simulink model "RTOS_Mail_blocking_Blinky"  (R2016b)
settings: Solver=FixedStepDiscrete  StartTime=0.0  StopTime=10.0  FixedStep=1e-3  RelTol=1e-3
libraries: mbed_lib x6
settings Model: MbedPath=E:\GitSynology\mbed_target\targets\NUCLEO_F303RE  Creator=oh  LastModifiedBy=oh
settings DataIOCC: LimitDataPoints=on  SaveFormat=Array
settings OptimizationCC: LifeSpan=1
settings DebuggingCC: SolverPrmCheckMsg=warning  SFUnexpectedBacktrackingDiag=warning  SFNoUnconditionalDefaultTransitionDiag=warning  SFExecutionAtInitializationDiag=none
settings HardwareCC: ProdBitPerPointer=32  ProdBitPerSizeT=32  ProdBitPerPtrDiffT=32  ProdLargestAtomicInteger=Long  ProdLargestAtomicFloat=Double  ProdIntDivRoundTo=Undefined  ProdWordSize=32  ProdHWDeviceType=ARM Compatible->ARM Cortex
settings ModelReferenceCC: PropagateSignalLabelsOutOfModel=off
settings RTWCC: SystemTargetFile=mbed.tlc  TemplateMakefile=mbed.tmf  Description=Mbed Target (Embedded Target)  TargetLang=C++
settings CodeAppCC: IgnoreCustomStorageClasses=off
settings STFCustomTargetCC: TargetLibSuffix=.a  GenerateSampleERTMain=on  CombineOutputUpdateFcns=on  ERTCustomFileBanners=on  SupportContinuousTime=off  SupportNonInlinedSFcns=off  RemoveResetFunc=on  MATLABClassNameForMDSCustomization=Simulink.SoftwareTarget.ERTCustomization  GRTInterface=off  SystemTargetFile=mbed.tlc
settings ERTTargetCC: GenerateSampleERTMain=on  ParMdlRefBuildCompliant=off  CompOptLevelCompliant=off  ConcurrentExecutionCompliant=off  ERTFirstTimeCompliant=off  ModelStepFunctionPrototypeControlCompliant=off  CPPClassGenCompliant=off  UseToolchainInfoCompliant=off  ERTCustomFileTemplate=mbed_file_process.tlc  ConvertIfToSwitch=off  SuppressUnreachableDefaultCases=off
settings ConfigComp: CovMetricSettings=dw  CovHtmlReporting=on  CovSaveCumulativeToWorkspaceVar=on  CovSaveSingleToWorkspaceVar=on  CovExternalEMLEnable=off  CovSFcnEnable=off

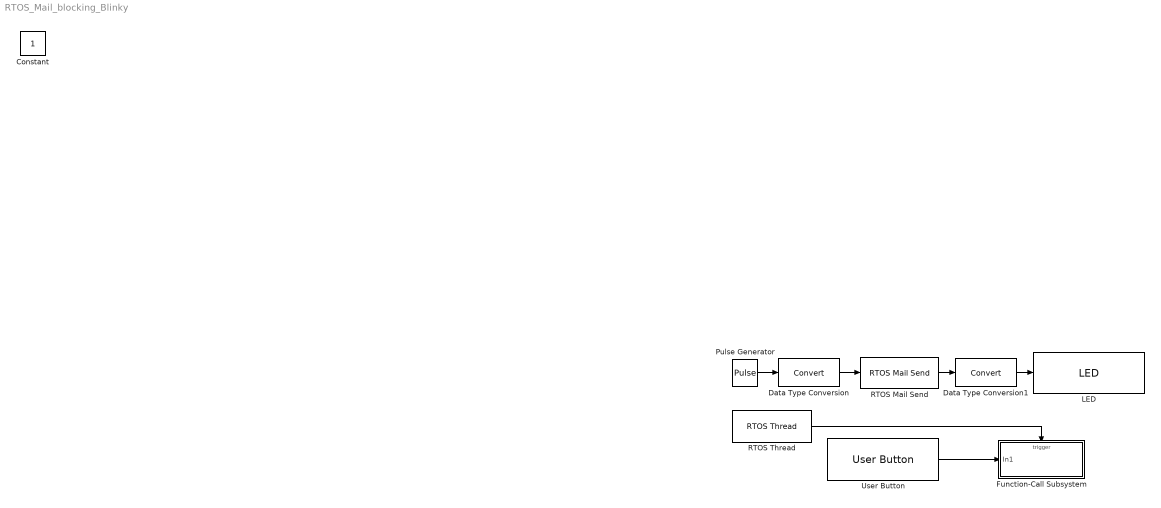
== system RTOS_Mail_blocking_Blinky ==
  Data Type Conversion : DataTypeConversion
  Data Type Conversion1 : DataTypeConversion
  Function-Call Subsystem : Subsystem  TreatAsAtomicUnit=on
  LED : mbed_lib/GPIO/LED  nLED=2  SampleTime=-1
  Pulse Generator : DiscretePulseGenerator  PulseType=Time based  Period=1  PulseWidth=20
  RTOS Mail Send : mbed_lib/RTOS/RTOS Mail Send  MailNumber=1  Timeout=1000  Depth=50  NumElements=1  DataType=uint8  EnableError=on
  RTOS Thread : mbed_lib/RTOS/RTOS Thread  ThreadPriority=Normal  StackOption=Default  StackSize=0  Timing=0
  User Button : mbed_lib/GPIO/User Button  SampleTime=0.1
  Constant : Constant  IOType=siggen
  wires:
  Pulse Generator/1 -> Data Type Conversion/1
  Data Type Conversion/1 -> RTOS Mail Send/1
  RTOS Mail Send/1 -> Data Type Conversion1/1
  Data Type Conversion1/1 -> LED/1
  RTOS Thread/1 -> Function-Call Subsystem/Trigger
  User Button/1 -> Function-Call Subsystem/1(In1)

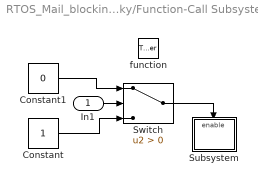
== system RTOS_Mail_blocking_Blinky/Function-Call Subsystem ==
  In1 : Inport
  function : TriggerPort  TriggerType=function-call  VariantControl=Variant
  Constant : Constant
  Constant1 : Constant  Value=0
  Subsystem : Subsystem
  Switch : Switch  Criteria=u2 > Threshold
  wires:
  In1/1 -> Switch/2
  Switch/1 -> Subsystem/Enable
  Constant1/1 -> Switch/1
  Constant/1 -> Switch/3

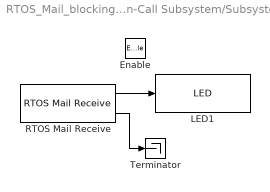
== system RTOS_Mail_blocking_Blinky/Function-Call Subsystem/Subsystem ==
  Enable : EnablePort
  LED1 : mbed_lib/GPIO/LED  nLED=1  SampleTime=-1
  RTOS Mail Receive : mbed_lib/RTOS/RTOS Mail Receive  MailNumber=1  Timeout=4294967295  NumElements=1  DataType=uint8
  Terminator : Terminator
  wires:
  RTOS Mail Receive/1 -> LED1/1
  RTOS Mail Receive/2 -> Terminator/1
